simulink model "animation"  (R2022a)
settings: Solver=VariableStepAuto  StartTime=0.0  StopTime=20  RelTol=1e-3
undefined symbols (not defined in the file or in its folder): car, disturb, E2TD, E2TN, T2VD
libraries: slpidlib x1
settings Model: Creator=Jirapu  LastModifiedBy=Jirapu

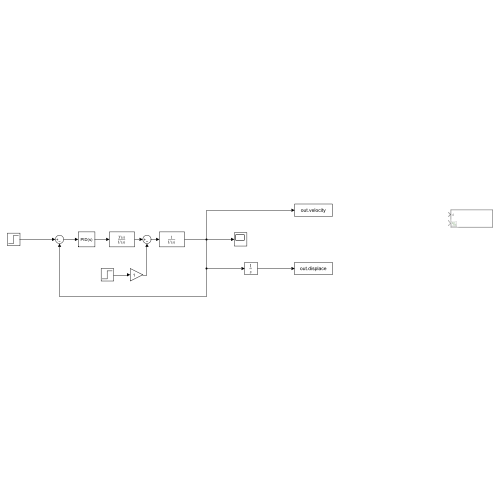
[thumbnail: Simulink's stored preview of the top-level diagram]
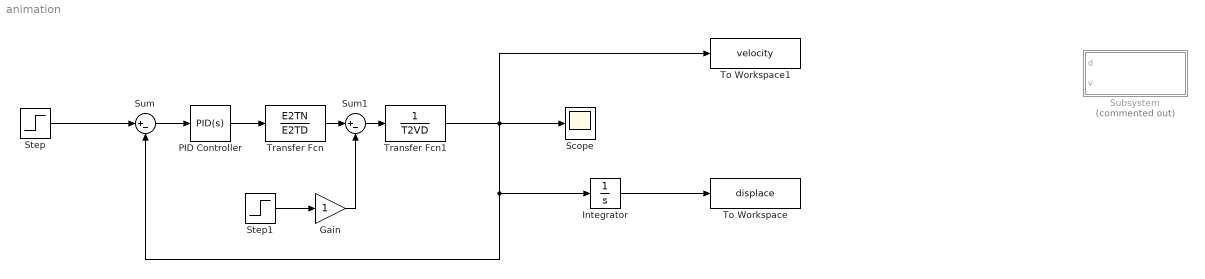
== system animation ==
  Gain : Gain
  Integrator : Integrator
  PID Controller : slpidlib/PID Controller  Controller=PID  Form=Parallel  TimeDomain=Continuous-time  UseExternalTs=off  SampleTime=-1  IntegratorMethod=Forward Euler  FilterMethod=Forward Euler  ControllerParametersSource=internal  P=30  I=60  UseKiTs=off  D=4  N=100  UseFilter=on  TunerSelectOption=Transfer Function Based (PID Tuner App)  InitialConditionSource=internal  InitialConditionForIntegrator=0  InitialConditionForFilter=0  DifferentiatorICPrevScaledInput=0  ExternalReset=none  TrackingMode=off  Kt=1  LimitOutput=off  SatLimitsSource=internal  UpperSaturationLimit=inf  LowerSaturationLimit=-inf  LinearizeAsGain=on  AntiWindupMode=none  Kb=1  POutMin=[]  POutMax=[]  IOutMin=[]  IOutMax=[]  DOutMin=[]  DOutMax=[]  NOutMin=[]  NOutMax=[]  SumOutMin=[]  SumOutMax=[]  SaturationOutMin=[]  SaturationOutMax=[]  PParamMin=[]  PParamMax=[]  IParamMin=[]  IParamMax=[]  DParamMin=[]  DParamMax=[]  NParamMin=[]  NParamMax=[]  KbParamMin=[]  KbParamMax=[]  KtParamMin=[]  KtParamMax=[]  KbOutMin=[]  KbOutMax=[]  KtOutMin=[]  KtOutMax=[]  IntegratorOutMin=[]  IntegratorOutMax=[]  FilterOutMin=[]  FilterOutMax=[]  SumI1OutMin=[]  SumI1OutMax=[]  SumI2OutMin=[]  SumI2OutMax=[]  SumI3OutMin=[]  SumI3OutMax=[]  SumI4OutMin=[]  SumI4OutMax=[]  SumDOutMin=[]  SumDOutMax=[]  DifferentiatorOutMin=[]  DifferentiatorOutMax=[]  FilterDiffOutCoefMin=[]  FilterDiffOutCoefMax=[]  ReciprocalOutMin=[]  ReciprocalOutMax=[]  SumDenOutMin=[]  SumDenOutMax=[]  SumNumOutMin=[]  SumNumOutMax=[]  DivideOutMin=[]  DivideOutMax=[]  UdiffTsProdOutMin=[]  UdiffTsProdOutMax=[]  NTsProdOutMin=[]  NTsProdOutMax=[]  UintegralTsProdOutMin=[]  UintegralTsProdOutMax=[]  UngainTsProdOutMin=[]  UngainTsProdOutMax=[]  IntegratorContinuousStateAttributes=''  IntegratorStateMustResolveToSignalObject=off  IntegratorRTWStateStorageClass=Auto  FilterContinuousStateAttributes=''  FilterStateMustResolveToSignalObject=off  FilterRTWStateStorageClass=Auto  ParallelPVariant=InternalParameters  IdealPVariant=Disabled  IVariant=InternalParameters  DVariant=InternalParameters  IntegratorVariant=Continuous  SatVariant=Disabled  AWVariant=Passthrough  PCopyVariant=Disabled  TRVariant=Disabled  FdbkBlocksVariant=Forward  IdealPFdbkVariant=Disabled  SatFdbkVariant=Disabled  DerivativeFilterVariant=ContFilter  NVariant=InternalParameters  NCopyVariant=Disabled  FilterICVariant=InternalICsFilter  IntegratorICVariant=InternalICs  ExternalResetVariant=Disabled  TRSumVariant=Passthrough  SumFdbkVariant=Disabled  SumVariant=Sum_PID  TsampFilterVariant=InternalTs  TsampNgainVariant=Passthrough  TsampIntegralVariant=Passthrough  ExternalSaturationOutDataTypeStr=Inherit: Same as second input  aMode=0
  Scope : Scope
  Step : Step  Time=0  After=car.V_desire  SampleTime=0
  Step1 : Step  Time=0  After=disturb  SampleTime=0
  Subsystem : Subsystem  Commented=on  TreatAsAtomicUnit=on  SystemSampleTime=0.1
  Sum : Sum  Inputs=|+-
  Sum1 : Sum  Inputs=|+-
  To Workspace : ToWorkspace  VariableName=displace  SampleTime=-1
  To Workspace1 : ToWorkspace  VariableName=velocity  SampleTime=-1
  Transfer Fcn : TransferFcn  Numerator=E2TN  Denominator=E2TD
  Transfer Fcn1 : TransferFcn  Denominator=T2VD
  wires:
  PID Controller/1 -> Transfer Fcn/1
  Transfer Fcn1/1 -> To Workspace1/1, Integrator/1, Sum/2, Scope/1
  Transfer Fcn/1 -> Sum1/1
  Sum1/1 -> Transfer Fcn1/1
  Step1/1 -> Gain/1
  Gain/1 -> Sum1/2
  Sum/1 -> PID Controller/1
  Step/1 -> Sum/1
  Integrator/1 -> To Workspace/1

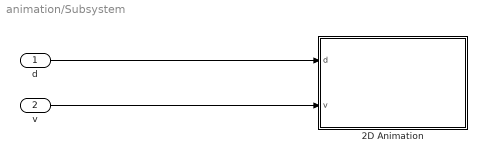
== system animation/Subsystem ==
  d : Inport
  v : Inport  Port=2
  2D Animation : MATLAB Function  TreatAsAtomicUnit=on
  wires:
  d/1 -> 2D Animation/1(d)
  v/1 -> 2D Animation/2(v)

== matlab function animation/Subsystem/2D Animation ==
  data: d input; v input
function plotVehicle(d,v)
cla;

x = d;
y = 0;
% car_Halflength = 2;
% car_Halfwidth = 1;
center = [x,y];
hold on
plot(x,y,"o")
hold off

% car_upper_x = linspace(center(1) - car_Halflength,center(1) + car_Halflength,10);
% car_upper_y = ones(10)*(center(2) + car_Halfwidth);
% car_lower_x = car_upper_x;
% car_lower_y = ones(10)*(center(2) - car_Halfwidth);
% car_left_x = ones(10)*(center(1) - car_Halflength);
% car_left_y = linspace(center(2) - car_Halfwidth,center(2) + car_Halfwidth,10);
% car_rigth_x = ones(10)*(center(1) + car_Halflength);
% car_rigth_y = car_left_y;

% plot car
% plot(car_upper_x,car_upper_y,"b-")
% plot(car_lower_x,car_lower_y,"b-")
% plot(car_left_x,car_left_y,"b-")
% plot(car_rigth_x,car_rigth_y,"b-")
% hold on
% plot(x,y,"o") % car center

% Road
% upperLine = plot([0 1000], [5 5], 'Color', 'blue');
% midLine = plot([0 1000], [0 0],'--', 'Color', 'blue');
% lowerLine = plot([0 1000], [-5 -5], 'Color', 'blue');
% hold off
% Velocity Display
disp(v)

% axis
% axis([center(1)-40 center(1)+40 center(2)-20 center(2)+20])
